simulink model "IP_LQG_PCI6221_2015a_Integrator"  (R2015a)
settings: Solver=ode3  StartTime=0.0  StopTime=200  RelTol=1e-3
values from neighbouring files (symbols this model uses):
  A = [A zeros(5,1) ... (first row only)    [IP_MACRO_Int_BEST.m]    (also in Integrador_Q_0d0001_gain_10_R_0d01.mat = [0 0 0 0 0 1 1 -0.0174048595758 0 -0.0173759205618 -232.0252; Integrador_Q_1.mat = [0 0 0 0 0 1 1 -0.0174048595758 0 -0.0173759205618 -232.0252; Q_1_0_100_0_0__R_0_1__Perturbacao.mat = [0 0 0 0 0 1 1 -0.0174048595758 0 -0.0173759205618 -232.0252; integrator.m)
  ALPHA_MAX = 90 * pi/180    (= 1.57079632679)    [IP_MACRO.m]    (also in IP_MACRO_Int_BEST.m; IP_MACRO_OP_TESTER.m; Integrador_Q_0d0001_gain_10_R_0d01.mat; Integrador_Q_1.mat)
  B = [B; 0]    [IP_MACRO_Int_BEST.m]    (also in Integrador_Q_0d0001_gain_10_R_0d01.mat = [0 0 0 0 333.33674813 0]; Integrador_Q_1.mat = [0 0 0 0 333.33674813 0]; Q_1_0_100_0_0__R_0_1__Perturbacao.mat = [0 0 0 0 333.33674813 0]; integrator.m)
  BETA_MAX = 15 * pi/180    (= 0.261799387799)    [IP_MACRO.m]    (also in IP_MACRO_Int_BEST.m; IP_MACRO_OP_TESTER.m; Integrador_Q_0d0001_gain_10_R_0d01.mat; Integrador_Q_1.mat)
  C = [1 0 0 0 0 0 ... (first row only)    [IP_MACRO_Int_BEST.m]    (also in Integrador_Q_0d0001_gain_10_R_0d01.mat = [1 0 0 0 0 0 0 1 0 0 0 0 ... (18 elements, 3x6)]; Integrador_Q_1.mat = [1 0 0 0 0 0 0 1 0 0 0 0 ... (18 elements, 3x6)]; Q_1_0_100_0_0__R_0_1__Perturbacao.mat = [1 0 0 0 0 0 0 1 0 0 0 0 ... (18 elements, 3x6)]; integrator.m)
  K = lqr(A, B, Qr, Rr)    [IP_MACRO.m]    (also in IP_MACRO_Int_BEST.m; IP_MACRO_OP_TESTER.m; Integrador_Q_0d0001_gain_10_R_0d01.mat = [-100.010598057 -34.2125648071 244.996893296 37.1465255495 0; Integrador_Q_1.mat = [-33.5897463141 -20.9783928184 205.877462394 31.1905076963 0)
  L = lqe(A, G, C, Qe, Re)    [IP_MACRO.m]    (also in IP_MACRO_Int_BEST.m; IP_MACRO_OP_TESTER.m = lqe(A, eye(size(A)), C, Qe, Re); Integrador_Q_0d0001_gain_10_R_0d01.mat = [3.22899659182 0.983246447527 1.1385177435 8.08815299126 -0.; Integrador_Q_1.mat = [3.22899659182 0.983246447527 1.1385177435 8.08815299126 -0.)
  TIME_DELAY = 6    [IP_MACRO.m]    (also in IP_MACRO_Int_BEST.m; IP_MACRO_OP_TESTER.m; Integrador_Q_0d0001_gain_10_R_0d01.mat; Integrador_Q_1.mat)
  Ts = 0.001    [IP_MACRO.m]    (also in IP_MACRO_Int_BEST.m; IP_MACRO_OP_TESTER.m; Integrador_Q_0d0001_gain_10_R_0d01.mat; Integrador_Q_1.mat)
  V_MAX = 5    [IP_MACRO.m]    (also in IP_MACRO_Int_BEST.m; IP_MACRO_OP_TESTER.m; Integrador_Q_0d0001_gain_10_R_0d01.mat; Integrador_Q_1.mat)
  V_MIN = -5    [IP_MACRO.m]    (also in IP_MACRO_Int_BEST.m; IP_MACRO_OP_TESTER.m; Integrador_Q_0d0001_gain_10_R_0d01.mat; Integrador_Q_1.mat)
undefined symbols (not defined in the file or in its folder): National_Instruments, PCI
libraries: sldrtlib x3, simulink x2
settings Model: SimulationMode=external  ExtModeTrigDuration=100000  Creator=Alunos  LastModifiedBy=Alunos
settings HardwareCC: ProdIntDivRoundTo=Zero  ProdEndianess=LittleEndian  ProdHWDeviceType=Intel->x86/Pentium  TargetIntDivRoundTo=Zero  TargetEndianess=LittleEndian  TargetHWDeviceType=Intel->x86/Pentium
settings RTWCC: SystemTargetFile=rtwin.tlc  TemplateMakefile=rtwin.tmf  Description=Simulink Desktop Real-Time  RTWCompilerOptimization=on
settings CodeAppCC: MaxIdLength=95
settings RTWinTargetCC: TargetPreCompLibLocation=C:\Program Files\MATLAB\R2015a\toolbox\sldrt\lib\win32

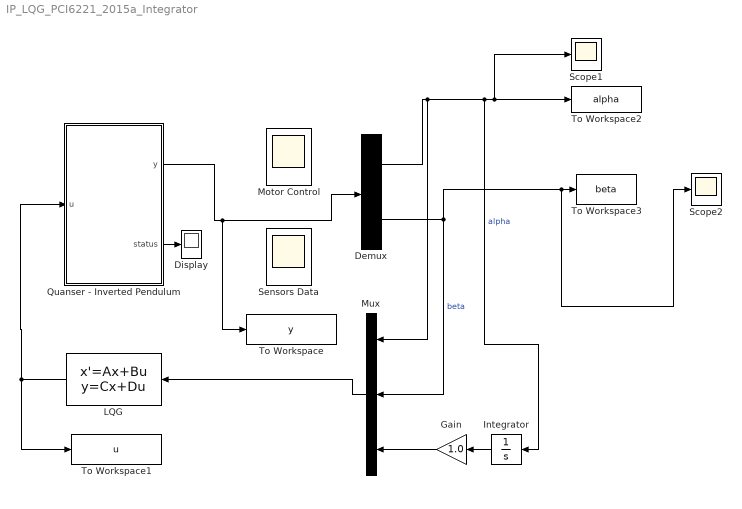
== system IP_LQG_PCI6221_2015a_Integrator ==
  Demux : Demux  Outputs=2
  Display : Display
  Gain : Gain  Gain=1.0
  Integrator : Integrator
  LQG : StateSpace  A=A-B*K-L*C  B=L  C=-K  D=zeros(1,3)  X0=0
  Motor Control : Scope
      settings: Floating=on  ShowLegends=on  SaveName=ScopeData2
  Mux : Mux  Inputs=3
  Quanser - Inverted Pendulum : Subsystem
      mask Display: image('IP_QUANSER.jpg');
  Scope1 : Scope
  Scope2 : Scope
      settings: YMin=-0.05  YMax=0.04  SaveName=ScopeData3
  Sensors Data : Scope
      settings: Floating=on  ShowLegends=on  YMin=-3.191592653589793  YMax=3.191592653589793
  To Workspace : ToWorkspace  VariableName=y  SampleTime=-1
  To Workspace1 : ToWorkspace  VariableName=u  SampleTime=-1
  To Workspace2 : ToWorkspace  VariableName=alpha  SampleTime=-1
  To Workspace3 : ToWorkspace  VariableName=beta  SampleTime=-1
  wires:
  LQG/1 -> Quanser - Inverted Pendulum/1(u), To Workspace1/1
  Quanser - Inverted Pendulum/2(status) -> Display/1
  Quanser - Inverted Pendulum/1(y) -> To Workspace/1, Demux/1
  Demux/2 -> Mux/2, Scope2/1, To Workspace3/1  "beta"
  Demux/1 -> Integrator/1, Scope1/1, To Workspace2/1, Mux/1  "alpha"
  Mux/1 -> LQG/1
  Integrator/1 -> Gain/1
  Gain/1 -> Mux/3

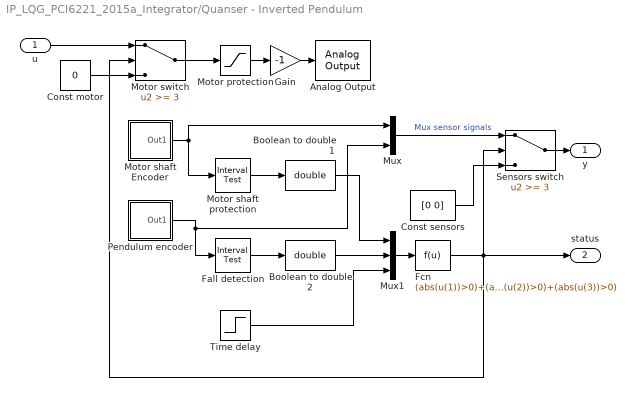
== system IP_LQG_PCI6221_2015a_Integrator/Quanser - Inverted Pendulum ==
  u : Inport
  Analog Output : sldrtlib/Analog Output  SampleTime=Ts  MaxMissedTicks=10  ShowMissedTicks=off  YieldWhenWaiting=off  DrvName=National_Instruments/PCI-6221  DrvAddress=4294967295  DrvOptions=[0 0 0 2 2]  Channels=1  RangeMode=1  VoltRange=1  InitialValue=0  FinalValue=0
      settings: AttributesFormatString=National Instruments\nPCI-6221 [auto]
  Boolean to double 1 : DataTypeConversion  OutDataTypeStr=double
  Boolean to double 2 : DataTypeConversion  OutDataTypeStr=double
  Const motor : Constant  Value=0
  Const sensors : Constant  Value=[0 0]
  Fall detection : simulink/Logic and Bit Operations/Interval Test  IntervalClosedRight=on  uplimit=BETA_MAX  IntervalClosedLeft=on  lowlimit=-BETA_MAX  OutDataTypeStr=uint8
  Fcn : Fcn  Expr=(abs(u(1))>0)+(abs(u(2))>0)+(abs(u(3))>0)
  Gain : Gain  Gain=-1
  Motor protection : Saturate  UpperLimit=V_MAX  LowerLimit=V_MIN
  Motor shaft Encoder : Subsystem
  Motor shaft protection : simulink/Logic and Bit Operations/Interval Test  IntervalClosedRight=on  uplimit=ALPHA_MAX  IntervalClosedLeft=on  lowlimit=-ALPHA_MAX  OutDataTypeStr=uint8
  Motor switch : Switch  Threshold=3
  Mux : Mux  Inputs=2
  Mux1 : Mux  Inputs=3
  Pendulum encoder : Subsystem
  Sensors switch : Switch  Threshold=3
  Time delay : Step  Time=TIME_DELAY  SampleTime=0
  y : Outport
  status : Outport  Port=2
  wires:
  u/1 -> Motor switch/1
  Motor switch/1 -> Motor protection/1
  Const motor/1 -> Motor switch/3
  Motor shaft Encoder/1(Out1) -> Mux/1, Motor shaft protection/1
  Pendulum encoder/1(Out1) -> Fall detection/1, Mux/2
  Mux1/1 -> Fcn/1
  Fcn/1 -> Sensors switch/2, status/1, Motor switch/2
  Time delay/1 -> Mux1/3
  Fall detection/1 -> Boolean to double 2/1
  Boolean to double 2/1 -> Mux1/2
  Motor shaft protection/1 -> Boolean to double 1/1
  Boolean to double 1/1 -> Mux1/1
  Const sensors/1 -> Sensors switch/3
  Mux/1 -> Sensors switch/1  "Mux sensor signals"
  Sensors switch/1 -> y/1
  Gain/1 -> Analog Output/1
  Motor protection/1 -> Gain/1

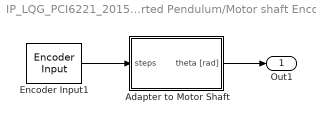
== system IP_LQG_PCI6221_2015a_Integrator/Quanser - Inverted Pendulum/Motor shaft Encoder ==
  Adapter to Motor Shaft : Subsystem
  Encoder Input1 : sldrtlib/Encoder Input  SampleTime=Ts  MaxMissedTicks=inf  ShowMissedTicks=off  YieldWhenWaiting=off  DrvName=National_Instruments/PCI-6221  DrvAddress=4294967295  DrvOptions=[0 0 0 2 2]  Channels=1  QuadMode=3  IndexPulse=2  InputFilter=Inf  DataType=1
      settings: AttributesFormatString=National Instruments\nPCI-6221 [auto]
  Out1 : Outport
  wires:
  Encoder Input1/1 -> Adapter to Motor Shaft/1(steps)
  Adapter to Motor Shaft/1(theta [rad]) -> Out1/1

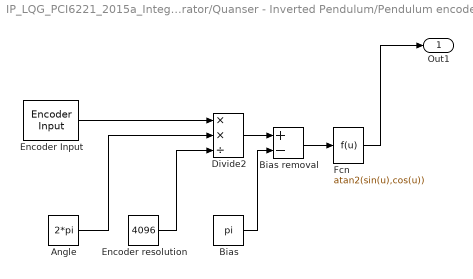
== system IP_LQG_PCI6221_2015a_Integrator/Quanser - Inverted Pendulum/Pendulum encoder ==
  Angle : Constant  Value=2*pi
  Bias : Constant  Value=pi
  Bias removal : Sum  Inputs=+-
  Divide2 : Product  Inputs=**/
  Encoder resolution : Constant  Value=4096
  Encoder Input : sldrtlib/Encoder Input  SampleTime=Ts  MaxMissedTicks=inf  ShowMissedTicks=off  YieldWhenWaiting=off  DrvName=National_Instruments/PCI-6221  DrvAddress=4294967295  DrvOptions=[0 0 0 2 2]  Channels=2  QuadMode=3  IndexPulse=2  InputFilter=Inf  DataType=1
      settings: AttributesFormatString=National Instruments\nPCI-6221 [auto]
  Fcn : Fcn  Expr=atan2(sin(u),cos(u))
  Out1 : Outport
  wires:
  Bias/1 -> Bias removal/2
  Encoder resolution/1 -> Divide2/3
  Divide2/1 -> Bias removal/1
  Fcn/1 -> Out1/1
  Encoder Input/1 -> Divide2/1
  Bias removal/1 -> Fcn/1
  Angle/1 -> Divide2/2

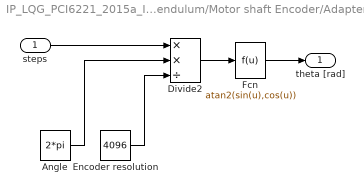
== system IP_LQG_PCI6221_2015a_Integrator/Quanser - Inverted Pendulum/Motor shaft Encoder/Adapter to Motor Shaft ==
  steps : Inport
  Angle : Constant  Value=2*pi
  Divide2 : Product  Inputs=**/
  Encoder resolution : Constant  Value=4096
  Fcn : Fcn  Expr=atan2(sin(u),cos(u))
  theta [rad] : Outport
  wires:
  Angle/1 -> Divide2/2
  Encoder resolution/1 -> Divide2/3
  steps/1 -> Divide2/1
  Divide2/1 -> Fcn/1
  Fcn/1 -> theta [rad]/1
